simulink model "linear_roll_control_R2015a"  (R2015b)
settings: Solver=ode45  StartTime=0.0  StopTime=10.0  RelTol=1e-3
values from neighbouring files (symbols this model uses):
  kda = [0]    [RunSimLab7.m]
  kdu = [0]    [RunSimLab7.m]    (also in RunSimLab7[Conflict].m)
  kia = [0]    [RunSimLab7.m]
  kiu = [0]    [RunSimLab7.m]    (also in RunSimLab7[Conflict].m = [.5])
  kpa = [0]    [RunSimLab7.m]
  kpr = [-7]    [RunSimLab7.m]    (also in RunSimLab7[Conflict].m)
  kpu = [0]    [RunSimLab7.m]    (also in RunSimLab7[Conflict].m = [.3])
  numP_r_from_dr = numPdr(3,:)    [RunSimLab7.m]    (also in RunSimLab7[Conflict].m)
  tau_w0 = -5    [RunSimLab7.m]
  yaw_com = 0.5*pi/180    (= 0.00872664625997)    [RunSimLab7.m]    (also in RunSimLab7[Conflict].m = 0.0872664625997)
undefined symbols (not defined in the file or in its folder): denPda, denPdr, numP_p_from_da, numP_p_from_dr, numP_phi_from_da, numP_phi_from_dr, numP_r_from_da, phi_com
libraries: dspsrcs4 x1
settings Model: Creator=Eric  LastModifiedBy=Jeremy
settings DataIOCC: SaveFormat=Array
settings OptimizationCC: ExpressionDepthLimit=2147483647
settings DebuggingCC: UnderspecifiedInitializationDetection=Classic  MergeDetectMultiDrivingBlocksExec=none  SolverPrmCheckMsg=warning  StateNameClashWarn=warning
settings HardwareCC: ProdBitPerPointer=32  ProdLargestAtomicFloat=None  ProdIntDivRoundTo=Undefined  ProdEndianess=Unspecified  ProdWordSize=32  ProdHWDeviceType=32-bit Generic
settings GRTTargetCC: GeneratePreprocessorConditionals=Disable all
settings ConfigComp: CovModelRefEnable=Off  CovSFcnEnable=off

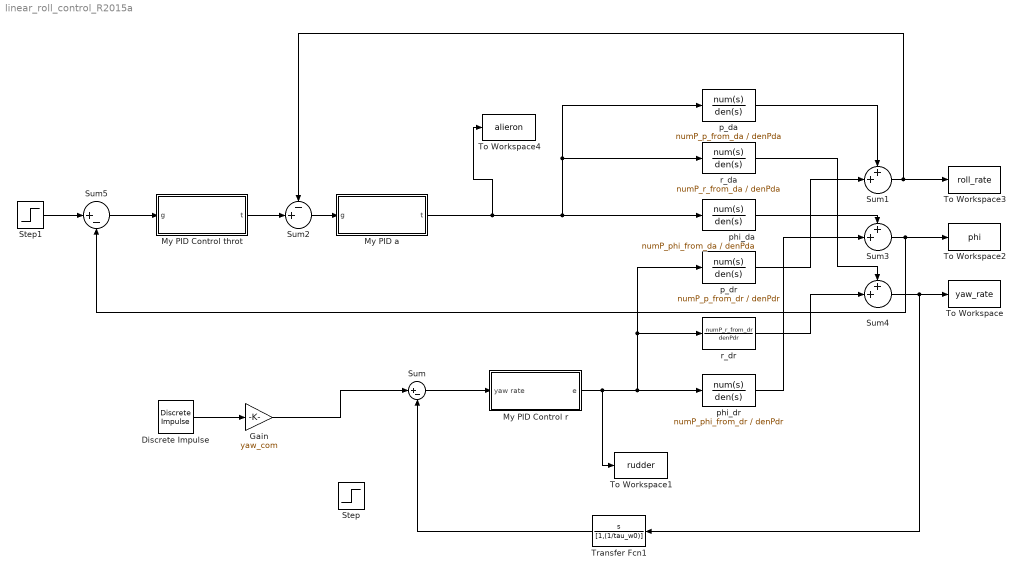
== system linear_roll_control_R2015a ==
  Discrete Impulse : dspsrcs4/Discrete  Impulse  Delay=1  SampleTime=1  FrameSample=1  OutputFrames=off  dataType=double  isSigned=on  wordLen=16  udDataType=sfix(16)  fracBitsMode=Best precision  numFracBits=15  OutDataTypeStr=double  LastOutDataTypeStr=double
  Gain : Gain  Gain=yaw_com
  My PID Control r : Subsystem  TreatAsAtomicUnit=on
  My PID Control throt : Subsystem  TreatAsAtomicUnit=on
  My PID a : Subsystem  TreatAsAtomicUnit=on
  Step : Step  Time=0  After=0  SampleTime=0
  Step1 : Step  Time=0  After=phi_com  SampleTime=0
  Sum : Sum  Inputs=|+-
  Sum1 : Sum  Inputs=++|
  Sum2 : Sum  Inputs=-+|
  Sum3 : Sum  Inputs=++|
  Sum4 : Sum  Inputs=++|
  Sum5 : Sum  Inputs=|+-
  To Workspace : ToWorkspace  VariableName=yaw_rate  SaveFormat=Timeseries  SampleTime=-1
  To Workspace1 : ToWorkspace  VariableName=rudder  SaveFormat=Timeseries  SampleTime=-1
  To Workspace2 : ToWorkspace  VariableName=phi  SaveFormat=Timeseries  SampleTime=-1
  To Workspace3 : ToWorkspace  VariableName=roll_rate  SaveFormat=Timeseries  SampleTime=-1
  To Workspace4 : ToWorkspace  VariableName=alieron  SaveFormat=Timeseries  SampleTime=-1
  Transfer Fcn1 : TransferFcn  Numerator=[1,0]  Denominator=[1,(1/tau_w0)]
  p_da : TransferFcn  Numerator=numP_p_from_da  Denominator=denPda
  p_dr : TransferFcn  Numerator=numP_p_from_dr  Denominator=denPdr
  phi_da : TransferFcn  Numerator=numP_phi_from_da  Denominator=denPda
  phi_dr : TransferFcn  Numerator=numP_phi_from_dr  Denominator=denPdr
  r_da : TransferFcn  Numerator=numP_r_from_da  Denominator=denPda
  r_dr : TransferFcn  Numerator=numP_r_from_dr  Denominator=denPdr
  wires:
  Sum/1 -> My PID Control r/1(yaw rate)
  My PID Control r/1(e) -> To Workspace1/1, r_dr/1, p_dr/1, phi_dr/1
  Transfer Fcn1/1 -> Sum/2
  Sum1/1 -> To Workspace3/1, Sum2/1
  Sum3/1 -> To Workspace2/1, Sum5/2
  Sum4/1 -> Transfer Fcn1/1, To Workspace/1
  p_da/1 -> Sum1/1
  p_dr/1 -> Sum1/2
  r_da/1 -> Sum4/1
  r_dr/1 -> Sum4/2
  phi_da/1 -> Sum3/1
  phi_dr/1 -> Sum3/2
  Step1/1 -> Sum5/1
  My PID a/1(t) -> To Workspace4/1, r_da/1, p_da/1, phi_da/1
  My PID Control throt/1(t) -> Sum2/2
  Sum2/1 -> My PID a/1(g)
  Sum5/1 -> My PID Control throt/1(g)
  Discrete Impulse/1 -> Gain/1
  Gain/1 -> Sum/1

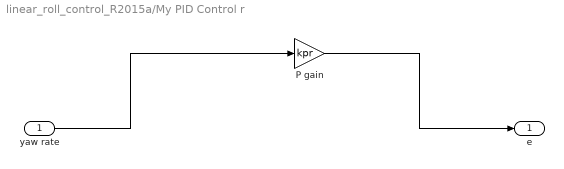
== system linear_roll_control_R2015a/My PID Control r ==
  yaw rate : Inport
  P gain : Gain  Gain=kpr
  e : Outport
  wires:
  yaw rate/1 -> P gain/1
  P gain/1 -> e/1

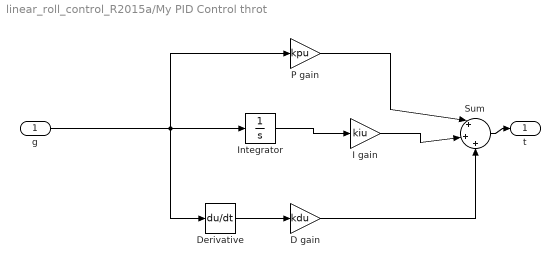
== system linear_roll_control_R2015a/My PID Control throt ==
  g : Inport
  D gain : Gain  Gain=kdu
  Derivative : Derivative
  I gain : Gain  Gain=kiu
  Integrator : Integrator
  P gain : Gain  Gain=kpu
  Sum : Sum  Inputs=|+|+|+
  t : Outport
  wires:
  g/1 -> Integrator/1, Derivative/1, P gain/1
  P gain/1 -> Sum/1
  Sum/1 -> t/1
  Derivative/1 -> D gain/1
  Integrator/1 -> I gain/1
  D gain/1 -> Sum/3
  I gain/1 -> Sum/2

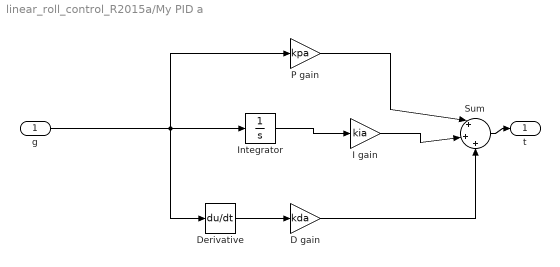
== system linear_roll_control_R2015a/My PID a ==
  g : Inport
  D gain : Gain  Gain=kda
  Derivative : Derivative
  I gain : Gain  Gain=kia
  Integrator : Integrator
  P gain : Gain  Gain=kpa
  Sum : Sum  Inputs=|+|+|+
  t : Outport
  wires:
  g/1 -> Integrator/1, Derivative/1, P gain/1
  P gain/1 -> Sum/1
  Sum/1 -> t/1
  Derivative/1 -> D gain/1
  Integrator/1 -> I gain/1
  D gain/1 -> Sum/3
  I gain/1 -> Sum/2
